simulink model "Model"  (R2024b)
settings: Solver=ode45  StartTime=0.0  StopTime=10  RelTol=1e-3
InitFcn:
  | Design
undefined symbols (not defined in the file): daq, drv, dspblkCoreblockFVToolHelper, DTF, ElecDyn, gbox, gcbh, ITF, Kd, Ki, Kp, MechDyn, mot, rads2rpm, Ref, sens, Tau_sf, Ts
libraries: simulink_extras x3
settings Model: Creator=Banaan  LastModifiedBy=Banaan

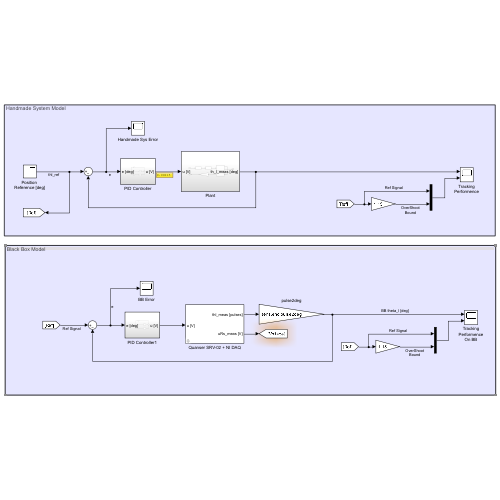
[thumbnail: Simulink's stored preview of the top-level diagram]
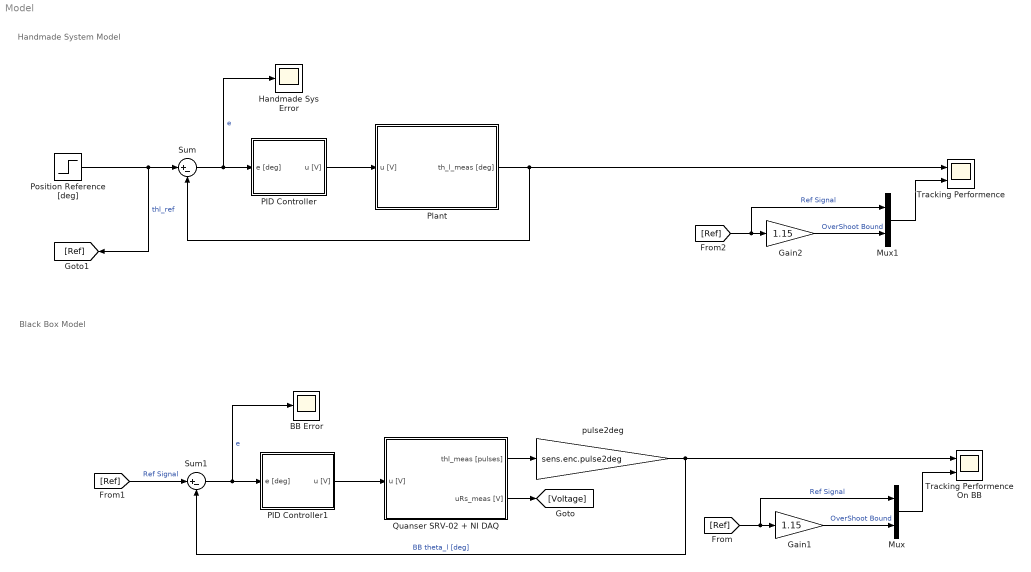
== system Model ==
  note: Handmade System Model
  note: Black Box Model
  BB Error : Scope
  Gain1 : Gain  Gain=1.15
  Gain2 : Gain  Gain=1.15
  Handmade Sys Error : Scope
  Mux : Mux  Inputs=2
  Mux1 : Mux  Inputs=2
  PID Controller : Subsystem
  PID Controller1 : Subsystem
  Plant : Subsystem
  Position Reference [deg] : Step  After=Ref  SampleTime=0
  Quanser SRV-02 + NI DAQ : Subsystem  mask(Quanser SRV-02 (with inertial load) + NI DAQ){Ts=0.001, fricType=Coulomb + viscous}
      mask prompts: Ts "NI DAQ Sample Time:"; fricType "Friction model"
      mask help: Quanser SRV-02 (with inertial load) + NI DAQ model.
      mask init:
      | %%  Sensors data
      | 
      | %   shunt resistor
      | sens.curr.Rs = 0.5;                         %   resistance [Ohm]   
      | sens.curr.uRs_std = 0.01;                   %   voltage noise standard dev [V]                           
      | sens.curr.uRs_var = sens.curr.uRs_std^2;	%   voltage noise variance [V^2]
      | 
      | %   Hewlett-Packard HEDS-5540#A06 optical encoder
      | sens.enc.ppr = 500*4;                       %   pulses per rotation
      | sens.enc.pulse2deg = 360/sens.enc.ppr;      %   [pulses] -> [deg]
      | sens.enc.pulse2rad = 2*pi/sens.enc.ppr;     %   [pulses] -> [rad]
      | sens.enc.deg2pulse = sens.enc.ppr/360;      %   [deg] -> [pulses]
      | sens.enc.rad2pulse = sens.enc.ppr/2/pi;     %   [rad] -> [pulses]
      | 
      | 
      | %%  Data acquisition board (daq) data
      | 
      | %   NI PCI-6221 DAC data
      | daq.dac.bits = 16;                                  %   resolution (bits)
      | daq.dac.fs   = 10;                                  %   full scale 
      | daq.dac.q    = 2*daq.dac.fs/(2^daq.dac.bits-1);     %	quantization
      | 
      | %   NI PCI-6221 ADC data
      | daq.adc.bits = 16;                                  %   resolution (bits)
      | daq.adc.fs   = 10;                                  %   full scale (as set in SLDRT Analog Input block)
      | daq.adc.q    = 2*daq.adc.fs/(2^daq.adc.bits-1);     %   quantization
      mask Help:
      | Riccardo Antonello (antonello@dei.unipd.it)
      | 
      | April 24, 2020
      | 
      | Dept. of Information Engineering, University of Padova
      mask TypeOptions fricType: Coulomb + viscous | Karnopp
  Sum : Sum  Inputs=|+-
  Sum1 : Sum  Inputs=|+-
  Tracking Performence : Scope  NumInputPorts=2
  Tracking Performence On BB : Scope  NumInputPorts=2
  pulse2deg : Gain  Gain=sens.enc.pulse2deg
  wires:
  PID Controller/1(u [V]) -> Plant/1(u [V])
  Sum/1 -> Handmade Sys Error/1, PID Controller/1(e [deg])  "e"
  Plant/1(th_l_meas [deg]) -> Tracking Performence/1, Sum/2
  Position Reference [deg]/1 -> [Ref], Sum/1  "thl_ref"
  Quanser SRV-02 + NI DAQ/1(thl_meas [pulses]) -> pulse2deg/1
  pulse2deg/1 -> Sum1/2, Tracking Performence On BB/1  "BB theta_l [deg]"
  Quanser SRV-02 + NI DAQ/2(uRs_meas [V]) -> [Voltage]
  Sum1/1 -> PID Controller1/1(e [deg]), BB Error/1  "e"
  PID Controller1/1(u [V]) -> Quanser SRV-02 + NI DAQ/1(u [V])
  Gain1/1 -> Mux/2  "OverShoot Bound"
  [Ref] -> Mux/1, Gain1/1  "Ref Signal"
  Mux/1 -> Tracking Performence On BB/2
  [Ref] -> Sum1/1  "Ref Signal"
  Mux1/1 -> Tracking Performence/2
  [Ref] -> Gain2/1, Mux1/1  "Ref Signal"
  Gain2/1 -> Mux1/2  "OverShoot Bound"

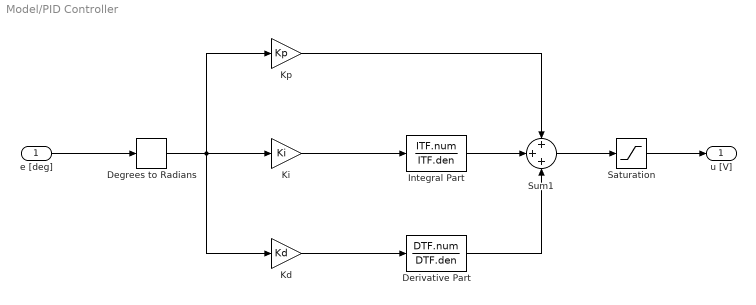
== system Model/PID Controller ==
  e [deg] : Inport
  Degrees to Radians : simulink_extras/Transformations/Degrees to Radians
  Derivative Part : DiscreteTransferFcn  LoadFcn=dspblkCoreblockFVToolHelper(gcbh,'load');  Numerator=DTF.num  Denominator=DTF.den  SampleTime=Ts
      settings: CopyFcn=dspblkCoreblockFVToolHelper(gcbh,'copy');  DeleteFcn=dspblkCoreblockFVToolHelper(gcbh,'close');  ModelCloseFcn=dspblkCoreblockFVToolHelper(gcbh,'close');  PreSaveFcn=dspblkCoreblockFVToolHelper(gcbh,'presave');  PostSaveFcn=dspblkCoreblockFVToolHelper(gcbh,'postsave');  CloseFcn=dspblkCoreblockFVToolHelper(gcbh,'close');
  Integral Part : DiscreteTransferFcn  LoadFcn=dspblkCoreblockFVToolHelper(gcbh,'load');  Numerator=ITF.num  Denominator=ITF.den  SampleTime=Ts
      settings: CopyFcn=dspblkCoreblockFVToolHelper(gcbh,'copy');  DeleteFcn=dspblkCoreblockFVToolHelper(gcbh,'close');  ModelCloseFcn=dspblkCoreblockFVToolHelper(gcbh,'close');  PreSaveFcn=dspblkCoreblockFVToolHelper(gcbh,'presave');  PostSaveFcn=dspblkCoreblockFVToolHelper(gcbh,'postsave');  CloseFcn=dspblkCoreblockFVToolHelper(gcbh,'close');
  Kd : Gain  Gain=Kd
  Ki : Gain  Gain=Ki
  Kp : Gain  Gain=Kp
  Saturation : Saturate  UpperLimit=daq.adc.fs  LowerLimit=-daq.adc.fs
  Sum1 : Sum  Inputs=+++
  u [V] : Outport
  wires:
  Degrees to Radians/1 -> Kd/1, Ki/1, Kp/1
  Derivative Part/1 -> Sum1/3
  Integral Part/1 -> Sum1/2
  Kd/1 -> Derivative Part/1
  Ki/1 -> Integral Part/1
  Kp/1 -> Sum1/1
  Sum1/1 -> Saturation/1
  e [deg]/1 -> Degrees to Radians/1
  Saturation/1 -> u [V]/1

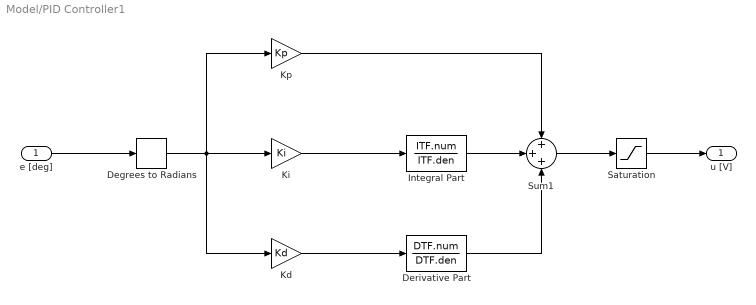
== system Model/PID Controller1 ==
  e [deg] : Inport
  Degrees to Radians : simulink_extras/Transformations/Degrees to Radians
  Derivative Part : DiscreteTransferFcn  LoadFcn=dspblkCoreblockFVToolHelper(gcbh,'load');  Numerator=DTF.num  Denominator=DTF.den  SampleTime=Ts
      settings: CopyFcn=dspblkCoreblockFVToolHelper(gcbh,'copy');  DeleteFcn=dspblkCoreblockFVToolHelper(gcbh,'close');  ModelCloseFcn=dspblkCoreblockFVToolHelper(gcbh,'close');  PreSaveFcn=dspblkCoreblockFVToolHelper(gcbh,'presave');  PostSaveFcn=dspblkCoreblockFVToolHelper(gcbh,'postsave');  CloseFcn=dspblkCoreblockFVToolHelper(gcbh,'close');
  Integral Part : DiscreteTransferFcn  LoadFcn=dspblkCoreblockFVToolHelper(gcbh,'load');  Numerator=ITF.num  Denominator=ITF.den  SampleTime=Ts
      settings: CopyFcn=dspblkCoreblockFVToolHelper(gcbh,'copy');  DeleteFcn=dspblkCoreblockFVToolHelper(gcbh,'close');  ModelCloseFcn=dspblkCoreblockFVToolHelper(gcbh,'close');  PreSaveFcn=dspblkCoreblockFVToolHelper(gcbh,'presave');  PostSaveFcn=dspblkCoreblockFVToolHelper(gcbh,'postsave');  CloseFcn=dspblkCoreblockFVToolHelper(gcbh,'close');
  Kd : Gain  Gain=Kd
  Ki : Gain  Gain=Ki
  Kp : Gain  Gain=Kp
  Saturation : Saturate  UpperLimit=daq.adc.fs  LowerLimit=-daq.adc.fs
  Sum1 : Sum  Inputs=+++
  u [V] : Outport
  wires:
  Derivative Part/1 -> Sum1/3
  Kd/1 -> Derivative Part/1
  Saturation/1 -> u [V]/1
  Kp/1 -> Sum1/1
  Degrees to Radians/1 -> Kd/1, Ki/1, Kp/1
  e [deg]/1 -> Degrees to Radians/1
  Ki/1 -> Integral Part/1
  Integral Part/1 -> Sum1/2
  Sum1/1 -> Saturation/1

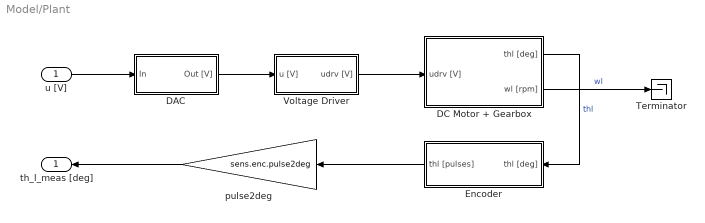
== system Model/Plant ==
  u [V] : Inport
  DAC : Subsystem
  DC Motor + Gearbox : Subsystem
  Encoder : Subsystem
  Terminator : Terminator
  Voltage Driver : Subsystem
  pulse2deg : Gain  Gain=sens.enc.pulse2deg
  th_l_meas [deg] : Outport
  wires:
  DAC/1(Out [V]) -> Voltage Driver/1(u [V])
  Encoder/1(thl [pulses]) -> pulse2deg/1
  u [V]/1 -> DAC/1(In)
  Voltage Driver/1(udrv [V]) -> DC Motor + Gearbox/1(udrv [V])
  DC Motor + Gearbox/2(wl [rpm]) -> Terminator/1  "wl"
  DC Motor + Gearbox/1(thl [deg]) -> Encoder/1(thl [deg])  "thl"
  pulse2deg/1 -> th_l_meas [deg]/1

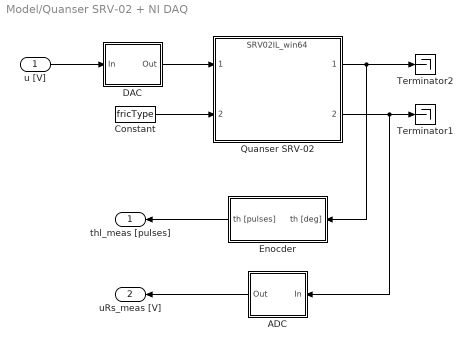
== system Model/Quanser SRV-02 + NI DAQ ==
  u [V] : Inport
  ADC : Subsystem
  Constant : Constant  Value=fricType
  DAC : Subsystem
  Enocder : Subsystem
  Quanser SRV-02 : ModelReference  ModelNameDialog=SRV02IL_win64.slxp  ModelReferenceVersion=1.44  CopyOfModelProtected=on
  Terminator1 : Terminator
  Terminator2 : Terminator
  thl_meas [pulses] : Outport
  uRs_meas [V] : Outport  Port=2
  wires:
  Enocder/1(th [pulses]) -> thl_meas [pulses]/1
  ADC/1(Out) -> uRs_meas [V]/1
  DAC/1(Out) -> Quanser SRV-02/1
  Quanser SRV-02/2 -> ADC/1(In), Terminator1/1
  u [V]/1 -> DAC/1(In)
  Quanser SRV-02/1 -> Enocder/1(th [deg]), Terminator2/1
  Constant/1 -> Quanser SRV-02/2

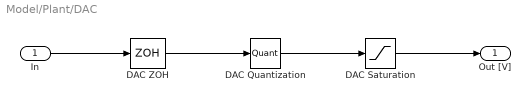
== system Model/Plant/DAC ==
  In : Inport
  DAC Quantization : Quantizer  QuantizationInterval=daq.dac.q
  DAC Saturation : Saturate  UpperLimit=daq.dac.fs  LowerLimit=-daq.dac.fs
  DAC ZOH : ZeroOrderHold  SampleTime=Ts
  Out [V] : Outport
  wires:
  DAC Quantization/1 -> DAC Saturation/1
  DAC ZOH/1 -> DAC Quantization/1
  DAC Saturation/1 -> Out [V]/1
  In/1 -> DAC ZOH/1

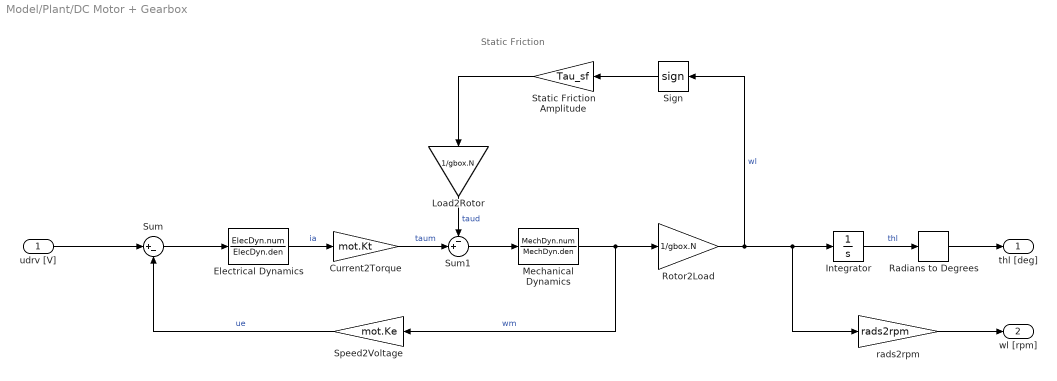
== system Model/Plant/DC Motor + Gearbox ==
  note: Static Friction
  udrv [V] : Inport
  Current2Torque : Gain  Gain=mot.Kt
  Electrical Dynamics : TransferFcn  Numerator=ElecDyn.num  Denominator=ElecDyn.den
  Integrator : Integrator
  Load2Rotor : Gain  Gain=1/gbox.N
  Mechanical Dynamics : TransferFcn  Numerator=MechDyn.num  Denominator=MechDyn.den
  Radians to Degrees : simulink_extras/Transformations/Radians to Degrees
  Rotor2Load : Gain  Gain=1/gbox.N
  Sign : Signum  ZeroCross=off
  Speed2Voltage : Gain  Gain=mot.Ke
  Static Friction Amplitude : Gain  Gain=Tau_sf
  Sum : Sum  Inputs=|+-
  Sum1 : Sum  Inputs=-+|
  rads2rpm : Gain  Gain=rads2rpm
  thl [deg] : Outport
  wl [rpm] : Outport  Port=2
  wires:
  Rotor2Load/1 -> rads2rpm/1, Integrator/1, Sign/1  "wl"
  Electrical Dynamics/1 -> Current2Torque/1  "ia"
  Sum1/1 -> Mechanical Dynamics/1
  Speed2Voltage/1 -> Sum/2  "ue"
  Load2Rotor/1 -> Sum1/1  "taud"
  Radians to Degrees/1 -> thl [deg]/1
  Mechanical Dynamics/1 -> Speed2Voltage/1, Rotor2Load/1  "wm"
  Sum/1 -> Electrical Dynamics/1
  Integrator/1 -> Radians to Degrees/1  "thl"
  Current2Torque/1 -> Sum1/2  "taum"
  rads2rpm/1 -> wl [rpm]/1
  Sign/1 -> Static Friction Amplitude/1
  Static Friction Amplitude/1 -> Load2Rotor/1
  udrv [V]/1 -> Sum/1

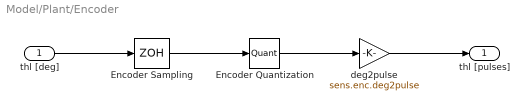
== system Model/Plant/Encoder ==
  thl [deg] : Inport
  Encoder Quantization : Quantizer  QuantizationInterval=daq.adc.q
  Encoder Sampling : ZeroOrderHold  SampleTime=Ts
  deg2pulse : Gain  Gain=sens.enc.deg2pulse
  thl [pulses] : Outport
  wires:
  Encoder Sampling/1 -> Encoder Quantization/1
  Encoder Quantization/1 -> deg2pulse/1
  thl [deg]/1 -> Encoder Sampling/1
  deg2pulse/1 -> thl [pulses]/1

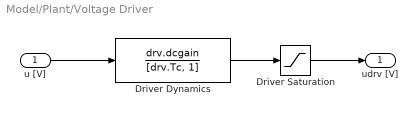
== system Model/Plant/Voltage Driver ==
  u [V] : Inport
  Driver Dynamics : TransferFcn  Numerator=drv.dcgain  Denominator=[drv.Tc, 1]
  Driver Saturation : Saturate  UpperLimit=drv.outmax  LowerLimit=-drv.outmax
  udrv [V] : Outport
  wires:
  Driver Dynamics/1 -> Driver Saturation/1
  u [V]/1 -> Driver Dynamics/1
  Driver Saturation/1 -> udrv [V]/1

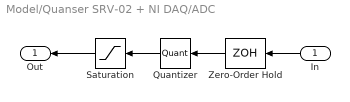
== system Model/Quanser SRV-02 + NI DAQ/ADC ==
  In : Inport
  Quantizer : Quantizer  QuantizationInterval=daq.adc.q
  Saturation : Saturate  UpperLimit=daq.adc.fs  LowerLimit=-daq.adc.fs
  Zero-Order Hold : ZeroOrderHold  SampleTime=Ts
  Out : Outport
  wires:
  Saturation/1 -> Out/1
  In/1 -> Zero-Order Hold/1
  Quantizer/1 -> Saturation/1
  Zero-Order Hold/1 -> Quantizer/1

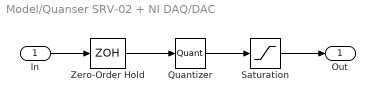
== system Model/Quanser SRV-02 + NI DAQ/DAC ==
  In : Inport
  Quantizer : Quantizer  QuantizationInterval=daq.dac.q
  Saturation : Saturate  UpperLimit=daq.dac.fs  LowerLimit=-daq.dac.fs
  Zero-Order Hold : ZeroOrderHold  SampleTime=Ts
  Out : Outport
  wires:
  Quantizer/1 -> Saturation/1
  In/1 -> Zero-Order Hold/1
  Zero-Order Hold/1 -> Quantizer/1
  Saturation/1 -> Out/1

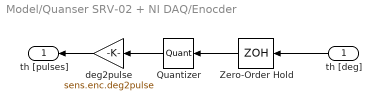
== system Model/Quanser SRV-02 + NI DAQ/Enocder ==
  th [deg] : Inport
  Quantizer : Quantizer  QuantizationInterval=sens.enc.pulse2deg
  Zero-Order Hold : ZeroOrderHold  SampleTime=Ts
  deg2pulse : Gain  Gain=sens.enc.deg2pulse
  th [pulses] : Outport
  wires:
  Quantizer/1 -> deg2pulse/1
  th [deg]/1 -> Zero-Order Hold/1
  Zero-Order Hold/1 -> Quantizer/1
  deg2pulse/1 -> th [pulses]/1
